simulink model "PreCondition"  (R2018b)
settings: Solver=FixedStepDiscrete  StartTime=0.0  StopTime=10.0  FixedStep=0.01  RelTol=1e-3
undefined symbols (not defined in the file or in its folder): EnergyMgLdShdRq1, HMI_2L_StMd10_Config_Val, HMI_2L_StMd11_Config_Val, HMI_2L_StMd12_Config_Val, HMI_2L_StMd13_Config_Val, HMI_2L_StMd14_Config_Val, HMI_2L_StMd15_Config_Val, HMI_2L_StMd16_Config_Val, HMI_2L_StMd17_Config_Val, HMI_2L_StMd18_Config_Val, HMI_2L_StMd19_Config_Val, HMI_2L_StMd1_Config_Val, HMI_2L_StMd20_Config_Val, HMI_2L_StMd21_Config_Val, HMI_2L_StMd22_Config_Val, HMI_2L_StMd23_Config_Val, HMI_2L_StMd24_Config_Val, HMI_2L_StMd25_Config_Val, HMI_2L_StMd26_Config_Val, HMI_2L_StMd27_Config_Val, HMI_2L_StMd28_Config_Val, HMI_2L_StMd29_Config_Val, HMI_2L_StMd2_Config_Val, HMI_2L_StMd30_Config_Val, HMI_2L_StMd31_Config_Val, HMI_2L_StMd32_Config_Val, HMI_2L_StMd3_Config_Val, HMI_2L_StMd4_Config_Val, HMI_2L_StMd5_Config_Val, HMI_2L_StMd6_Config_Val, HMI_2L_StMd7_Config_Val, HMI_2L_StMd8_Config_Val, HMI_2L_StMd9_Config_Val, HMI_2R_StMd10_Config_Val, HMI_2R_StMd11_Config_Val, HMI_2R_StMd12_Config_Val, HMI_2R_StMd13_Config_Val, HMI_2R_StMd14_Config_Val, HMI_2R_StMd15_Config_Val, HMI_2R_StMd16_Config_Val, HMI_2R_StMd17_Config_Val, HMI_2R_StMd18_Config_Val, HMI_2R_StMd19_Config_Val, HMI_2R_StMd1_Config_Val, HMI_2R_StMd20_Config_Val, HMI_2R_StMd21_Config_Val, HMI_2R_StMd22_Config_Val, HMI_2R_StMd23_Config_Val, HMI_2R_StMd24_Config_Val, HMI_2R_StMd25_Config_Val, HMI_2R_StMd26_Config_Val, HMI_2R_StMd27_Config_Val, HMI_2R_StMd28_Config_Val, HMI_2R_StMd29_Config_Val, HMI_2R_StMd2_Config_Val, HMI_2R_StMd30_Config_Val, HMI_2R_StMd31_Config_Val, HMI_2R_StMd32_Config_Val, HMI_2R_StMd3_Config_Val, HMI_2R_StMd4_Config_Val ... (+94)
(part 5 of 6)

== system PreCondition/PreConitionRunnable_sys/Subsystem3/AcsEntry4s2LMd ==
  CommCond : Inport
  AcsEntry4s2LMdConfig : Inport  Port=2
  SecRwLtStChldLkReq : Inport  Port=3
  AcsEntry4s2LPosLrnd : Inport  Port=4
  Is2LStSwAct : Inport  Port=5
  SecRwLtStPosRclRspStat : Inport  Port=6
  AND : Logic  Inputs=6  AllPortsSameDT=off  OutDataTypeStr=boolean
  Constant1 : Constant  Value=SeatChldLkSt.ChldLkSt_Unlock  OutDataTypeStr=Enum:SeatChldLkSt
  Constant4 : Constant  Value=PosRclRspStat1.PosRclRspStat_None  OutDataTypeStr=Enum:PosRclRspStat1
  Equal : RelationalOperator  Operator===  OutDataTypeStr=boolean  RndMeth=Simplest
  Equal5 : RelationalOperator  Operator===  OutDataTypeStr=boolean  RndMeth=Simplest
  NOT : Logic  Operator=NOT  AllPortsSameDT=off  OutDataTypeStr=boolean
  "AcsEntry4s2LAvl " : Outport
  wires:
  CommCond/1 -> AND/1
  AcsEntry4s2LMdConfig/1 -> AND/2
  AND/1 -> "AcsEntry4s2LAvl "/1
  AcsEntry4s2LPosLrnd/1 -> AND/4
  NOT/1 -> AND/5
  Is2LStSwAct/1 -> NOT/1
  Constant1/1 -> Equal5/2
  SecRwLtStChldLkReq/1 -> Equal5/1
  Equal5/1 -> AND/3
  Constant4/1 -> Equal/2
  [SecRwLtStPosRclRspStat] -> Equal/1
  Equal/1 -> AND/6
  SecRwLtStPosRclRspStat/1 -> [SecRwLtStPosRclRspStat]

== system PreCondition/PreConitionRunnable_sys/Subsystem3/AcsEntry4s2RMd ==
  CommCond : Inport
  AcsEntry4s2RMdConfig : Inport  Port=2
  SecRwRtStChldLkReq : Inport  Port=3
  AcsEntry4s2RPosLrnd : Inport  Port=4
  Is2RStSwAct : Inport  Port=5
  VeSignalLost2R_463_2L : Inport  Port=6
  SecRwRtStPosRclRspStat : Inport  Port=7
  AND : Logic  Inputs=7  AllPortsSameDT=off  OutDataTypeStr=boolean
  Constant3 : Constant  Value=SeatChldLkSt.ChldLkSt_Unlock  OutDataTypeStr=Enum:SeatChldLkSt
  Constant4 : Constant  Value=PosRclRspStat1.PosRclRspStat_None  OutDataTypeStr=Enum:PosRclRspStat1
  Equal : RelationalOperator  Operator===  OutDataTypeStr=boolean  RndMeth=Simplest
  Equal2 : RelationalOperator  Operator===  OutDataTypeStr=boolean  RndMeth=Simplest
  NOT : Logic  Operator=NOT  AllPortsSameDT=off  OutDataTypeStr=boolean
  NOT1 : Logic  Operator=NOT  AllPortsSameDT=off  OutDataTypeStr=boolean
  "AcsEntry4s2RAvl " : Outport
  wires:
  CommCond/1 -> AND/1
  AcsEntry4s2RMdConfig/1 -> AND/2
  AND/1 -> "AcsEntry4s2RAvl "/1
  AcsEntry4s2RPosLrnd/1 -> AND/4
  NOT/1 -> AND/5
  Is2RStSwAct/1 -> NOT/1
  VeSignalLost2R_463_2L/1 -> NOT1/1
  NOT1/1 -> AND/6
  Equal2/1 -> AND/3
  SecRwRtStChldLkReq/1 -> Equal2/1
  Constant3/1 -> Equal2/2
  Constant4/1 -> Equal/2
  [SecRwRtStPosRclRspStat] -> Equal/1
  Equal/1 -> AND/7
  SecRwRtStPosRclRspStat/1 -> [SecRwRtStPosRclRspStat]

== system PreCondition/PreConitionRunnable_sys/Subsystem3/AcsEntryAll4sBwdMd ==
  CommCond : Inport
  AcsEntryAll4sBwdMdConfig : Inport  Port=2
  SecRwLtStChldLkReq : Inport  Port=3
  SecRwRtStChldLkReq : Inport  Port=4
  AcsEntryAll4sBwdPosLrnd : Inport  Port=5
  Is2LStSwAct : Inport  Port=6
  Is2RStSwAct : Inport  Port=7
  VeSignalLost2R_463_2L : Inport  Port=8
  SecRwLtStPosRclRspStat : Inport  Port=9
  SecRwRtStPosRclRspStat : Inport  Port=10
  AND : Logic  Inputs=7  AllPortsSameDT=off  OutDataTypeStr=boolean
  AND1 : Logic  AllPortsSameDT=off  OutDataTypeStr=boolean
  AND2 : Logic  AllPortsSameDT=off  OutDataTypeStr=boolean
  Constant1 : Constant  Value=SeatChldLkSt.ChldLkSt_Unlock  OutDataTypeStr=Enum:SeatChldLkSt
  Constant2 : Constant  Value=PosRclRspStat1.PosRclRspStat_None  OutDataTypeStr=Enum:PosRclRspStat1
  Constant4 : Constant  Value=PosRclRspStat1.PosRclRspStat_None  OutDataTypeStr=Enum:PosRclRspStat1
  Equal{,1..2,5} (4 alike) : RelationalOperator  Operator===  OutDataTypeStr=boolean  RndMeth=Simplest
  NOT : Logic  Operator=NOT  AllPortsSameDT=off  OutDataTypeStr=boolean
  NOT1 : Logic  Operator=NOT  AllPortsSameDT=off  OutDataTypeStr=boolean
  OR : Logic  Operator=OR  AllPortsSameDT=off  OutDataTypeStr=boolean
  "AcsEntryAll4sBwdAvl " : Outport
  wires:
  OR/1 -> NOT/1
  Is2RStSwAct/1 -> OR/2
  Is2LStSwAct/1 -> OR/1
  Equal1/1 -> AND1/2
  SecRwRtStChldLkReq/1 -> Equal1/2
  SecRwLtStChldLkReq/1 -> Equal5/1
  Constant1/1 -> Equal5/2, Equal1/1
  AND1/1 -> AND/3
  Equal5/1 -> AND1/1
  NOT1/1 -> AND/6
  VeSignalLost2R_463_2L/1 -> NOT1/1
  NOT/1 -> AND/5
  AcsEntryAll4sBwdPosLrnd/1 -> AND/4
  AND/1 -> "AcsEntryAll4sBwdAvl "/1
  AcsEntryAll4sBwdMdConfig/1 -> AND/2
  CommCond/1 -> AND/1
  [SecRwRtStPosRclRspStat] -> Equal2/1
  Equal2/1 -> AND2/2
  Constant2/1 -> Equal2/2
  [SecRwLtStPosRclRspStat] -> Equal/1
  Constant4/1 -> Equal/2
  Equal/1 -> AND2/1
  AND2/1 -> AND/7
  SecRwLtStPosRclRspStat/1 -> [SecRwLtStPosRclRspStat]
  SecRwRtStPosRclRspStat/1 -> [SecRwRtStPosRclRspStat]

== system PreCondition/PreConitionRunnable_sys/Subsystem3/AcsEntryAll4sFwdMd ==
  CommCond : Inport
  AcsEntryAll4sFwdMdConfig : Inport  Port=2
  SecRwLtStChldLkReq : Inport  Port=3
  SecRwRtStChldLkReq : Inport  Port=4
  AcsEntryAll4sFwdPosLrnd : Inport  Port=5
  Is2LStSwAct : Inport  Port=6
  Is2RStSwAct : Inport  Port=7
  VeSignalLost2R_463_2L : Inport  Port=8
  SecRwLtStPosRclRspStat : Inport  Port=9
  SecRwRtStPosRclRspStat : Inport  Port=10
  AND : Logic  Inputs=7  AllPortsSameDT=off  OutDataTypeStr=boolean
  AND1 : Logic  AllPortsSameDT=off  OutDataTypeStr=boolean
  AND2 : Logic  AllPortsSameDT=off  OutDataTypeStr=boolean
  Constant1 : Constant  Value=SeatChldLkSt.ChldLkSt_Unlock  OutDataTypeStr=Enum:SeatChldLkSt
  Constant2 : Constant  Value=PosRclRspStat1.PosRclRspStat_None  OutDataTypeStr=Enum:PosRclRspStat1
  Constant4 : Constant  Value=PosRclRspStat1.PosRclRspStat_None  OutDataTypeStr=Enum:PosRclRspStat1
  Equal{,1..2,5} (4 alike) : RelationalOperator  Operator===  OutDataTypeStr=boolean  RndMeth=Simplest
  NOT : Logic  Operator=NOT  AllPortsSameDT=off  OutDataTypeStr=boolean
  NOT1 : Logic  Operator=NOT  AllPortsSameDT=off  OutDataTypeStr=boolean
  OR : Logic  Operator=OR  AllPortsSameDT=off  OutDataTypeStr=boolean
  "AcsEntryAll4sFwdAvl " : Outport
  wires:
  CommCond/1 -> AND/1
  AcsEntryAll4sFwdMdConfig/1 -> AND/2
  AND/1 -> "AcsEntryAll4sFwdAvl "/1
  AcsEntryAll4sFwdPosLrnd/1 -> AND/4
  NOT/1 -> AND/5
  VeSignalLost2R_463_2L/1 -> NOT1/1
  NOT1/1 -> AND/6
  Equal5/1 -> AND1/1
  AND1/1 -> AND/3
  Constant1/1 -> Equal1/1, Equal5/2
  SecRwLtStChldLkReq/1 -> Equal5/1
  SecRwRtStChldLkReq/1 -> Equal1/2
  Equal1/1 -> AND1/2
  Is2LStSwAct/1 -> OR/1
  Is2RStSwAct/1 -> OR/2
  OR/1 -> NOT/1
  Constant4/1 -> Equal/2
  [SecRwLtStPosRclRspStat] -> Equal/1
  Constant2/1 -> Equal2/2
  [SecRwRtStPosRclRspStat] -> Equal2/1
  Equal/1 -> AND2/1
  Equal2/1 -> AND2/2
  AND2/1 -> AND/7
  SecRwLtStPosRclRspStat/1 -> [SecRwLtStPosRclRspStat]
  SecRwRtStPosRclRspStat/1 -> [SecRwRtStPosRclRspStat]

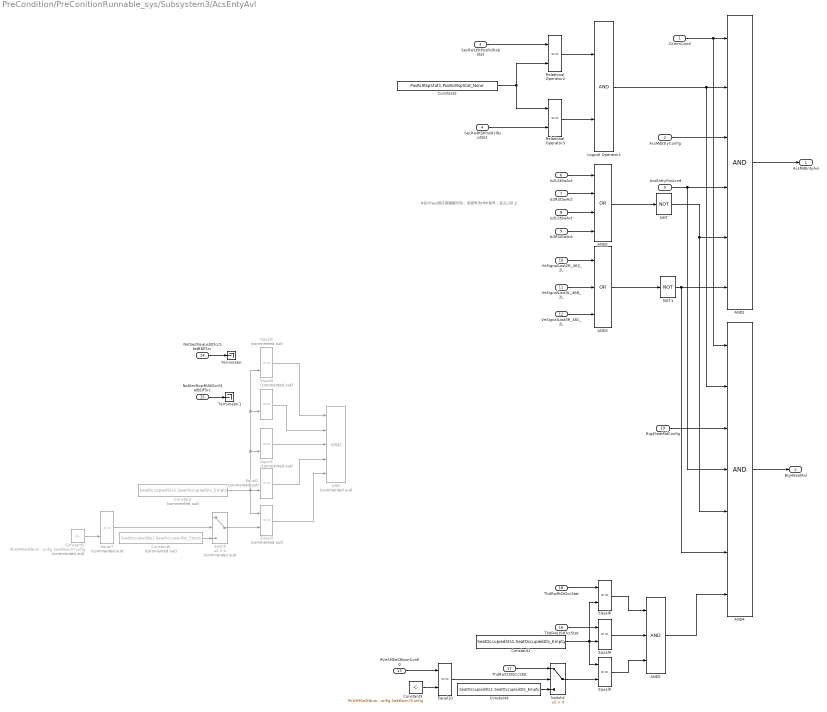
== system PreCondition/PreConitionRunnable_sys/Subsystem3/AcsEntyAvl ==
  note: #Dr/Pass侧只有脚蹬可动，该信号为HMI信号，在2L/2R上
  CommCond : Inport
  AcsMdEtryConfig : Inport  Port=2
  SecRwLtStPosRclRspStat : Inport  Port=3
  SecRwRtStPosRclRspStat : Inport  Port=4
  AcsEntryPosLrnd : Inport  Port=5
  Is2LStSwAct : Inport  Port=6
  Is2RStSwAct : Inport  Port=7
  Is3LStSwAct : Inport  Port=8
  Is3RStSwAct : Inport  Port=9
  VeSignalLost2R_463_2L : Inport  Port=10
  VeSignalLost3L_468_2L : Inport  Port=11
  VeSignalLost3R_46C_2L : Inport  Port=12
  IfVeSMSeStNumConfig : Inport  Port=13
  NotSecRowLeStOccStatBDFSrc : Inport  Port=14
  NotSecRowRtStOccStatBDFSrc : Inport  Port=15
  ThdRwLtStOccStat : Inport  Port=16
  ThdRwCtStOccStat : Inport  Port=17
  ThdRwRtStOccStat : Inport  Port=18
  Big4SeatMdConfig : Inport  Port=19
  AND : Logic  Commented=on  Inputs=5  AllPortsSameDT=off  OutDataTypeStr=boolean
  AND1 : Logic  Inputs=6  AllPortsSameDT=off  OutDataTypeStr=boolean
  AND2 : Logic  Operator=OR  Inputs=4  AllPortsSameDT=off  OutDataTypeStr=boolean
  AND3 : Logic  Operator=OR  Inputs=3  AllPortsSameDT=off  OutDataTypeStr=boolean
  AND4 : Logic  Inputs=7  AllPortsSameDT=off  OutDataTypeStr=boolean
  AND5 : Logic  Inputs=3  AllPortsSameDT=off  OutDataTypeStr=boolean
  Constant : Constant  Commented=on  Value=SeatOccupiedSts1.SeatOccupiedSts_Empty  OutDataTypeStr=Enum:SeatOccupiedSts1
  Constant1 : Constant  Value=SeatOccupiedSts1.SeatOccupiedSts_Empty  OutDataTypeStr=Enum:SeatOccupiedSts1
  Constant2 : Constant  Value=PosRclRspStat1.PosRclRspStat_None  OutDataTypeStr=Enum:PosRclRspStat1
  Constant3 : Constant  Value=IfVeSMSeStNumConfig.SeatNum7Config  OutDataTypeStr=Enum: IfVeSMSeStNumConfig
  Constant4 : Constant  Value=SeatOccupiedSts1.SeatOccupiedSts_Empty  OutDataTypeStr=Enum:SeatOccupiedSts1
  Constant5 : Constant  Commented=on  Value=IfVeSMSeStNumConfig.SeatNum7Config  OutDataTypeStr=Enum: IfVeSMSeStNumConfig
  Constant6 : Constant  Commented=on  Value=SeatOccupiedSts1.SeatOccupiedSts_Empty  OutDataTypeStr=Enum:SeatOccupiedSts1
  Equal{1..5,7} (6 alike) : RelationalOperator  Commented=on  Operator===  OutDataTypeStr=boolean  RndMeth=Simplest
  Equal{6,8..10} (4 alike) : RelationalOperator  Operator===  OutDataTypeStr=boolean  RndMeth=Simplest
  Logical Operator1 : Logic  AllPortsSameDT=off  OutDataTypeStr=boolean
  NOT : Logic  Operator=NOT  AllPortsSameDT=off  OutDataTypeStr=boolean
  NOT1 : Logic  Operator=NOT  AllPortsSameDT=off  OutDataTypeStr=boolean
  Relational Operator2 : RelationalOperator  Operator===  OutDataTypeStr=boolean  RndMeth=Simplest
  Relational Operator3 : RelationalOperator  Operator===  OutDataTypeStr=boolean  RndMeth=Simplest
  Switch : Switch  Commented=on  Criteria=u2 > Threshold
  Switch1 : Switch  Criteria=u2 > Threshold
  Terminator : Terminator
  Terminator1 : Terminator
  "AcsMdEntyAvl " : Outport
  Big4SeatAvl : Outport  Port=2
  wires:
  SecRwLtStPosRclRspStat/1 -> Relational Operator2/1
  Constant2/1 -> Relational Operator3/1, Relational Operator2/2
  Logical Operator1/1 -> AND4/2, AND1/2
  CommCond/1 -> AND4/1, AND1/1
  AcsMdEtryConfig/1 -> AND1/3
  AND1/1 -> "AcsMdEntyAvl "/1
  AND2/1 -> NOT/1
  AND3/1 -> NOT1/1
  AcsEntryPosLrnd/1 -> AND4/4, AND1/4
  NOT/1 -> AND4/5, AND1/5
  NOT1/1 -> AND4/6, AND1/6
  VeSignalLost2R_463_2L/1 -> AND3/1
  Relational Operator2/1 -> Logical Operator1/1
  Relational Operator3/1 -> Logical Operator1/2
  SecRwRtStPosRclRspStat/1 -> Relational Operator3/2
  Is2LStSwAct/1 -> AND2/1
  Is2RStSwAct/1 -> AND2/2
  Equal7/1 -> Switch/2
  Constant5/1 -> Equal7/2
  Constant/1 -> Equal5/2, Equal4/2, Equal1/2, Equal2/2, Equal3/1
  Constant6/1 -> Switch/3
  Switch/1 -> Equal3/2
  Equal1/1 -> AND/3
  Equal5/1 -> AND/1
  Equal4/1 -> AND/2
  Equal2/1 -> AND/4
  Equal3/1 -> AND/5
  VeSignalLost3R_46C_2L/1 -> AND3/3
  VeSignalLost3L_468_2L/1 -> AND3/2
  Is3RStSwAct/1 -> AND2/4
  Is3LStSwAct/1 -> AND2/3
  NotSecRowLeStOccStatBDFSrc/1 -> Terminator/1
  NotSecRowRtStOccStatBDFSrc/1 -> Terminator1/1
  Big4SeatMdConfig/1 -> AND4/3
  Equal10/1 -> Switch1/2
  Constant3/1 -> Equal10/2
  Constant1/1 -> Equal6/2, Equal8/2, Equal9/1
  Constant4/1 -> Switch1/3
  Switch1/1 -> Equal9/2
  IfVeSMSeStNumConfig/1 -> Equal10/1
  ThdRwCtStOccStat/1 -> Switch1/1
  ThdRwRtStOccStat/1 -> Equal6/1
  ThdRwLtStOccStat/1 -> Equal8/1
  Equal8/1 -> AND5/2
  Equal6/1 -> AND5/1
  Equal9/1 -> AND5/3
  AND5/1 -> AND4/7
  AND4/1 -> Big4SeatAvl/1

== system PreCondition/PreConitionRunnable_sys/Subsystem3/AcsExit4s2LMd ==
  CommCond : Inport
  AcsExit4s2LMdConfig : Inport  Port=2
  SecRwLtStChldLkReq : Inport  Port=3
  AcsExit4s2LPosLrnd : Inport  Port=4
  Is2LStSwAct : Inport  Port=5
  SecRwLtStPosRclRspStat : Inport  Port=6
  AND : Logic  Inputs=6  AllPortsSameDT=off  OutDataTypeStr=boolean
  Constant1 : Constant  Value=SeatChldLkSt.ChldLkSt_Unlock  OutDataTypeStr=Enum:SeatChldLkSt
  Constant4 : Constant  Value=PosRclRspStat1.PosRclRspStat_None  OutDataTypeStr=Enum:PosRclRspStat1
  Equal : RelationalOperator  Operator===  OutDataTypeStr=boolean  RndMeth=Simplest
  Equal5 : RelationalOperator  Operator===  OutDataTypeStr=boolean  RndMeth=Simplest
  NOT : Logic  Operator=NOT  AllPortsSameDT=off  OutDataTypeStr=boolean
  "AcsExit4s2LAvl " : Outport
  wires:
  Is2LStSwAct/1 -> NOT/1
  NOT/1 -> AND/5
  AcsExit4s2LPosLrnd/1 -> AND/4
  AND/1 -> "AcsExit4s2LAvl "/1
  AcsExit4s2LMdConfig/1 -> AND/2
  CommCond/1 -> AND/1
  SecRwLtStChldLkReq/1 -> Equal5/1
  Constant1/1 -> Equal5/2
  Equal5/1 -> AND/3
  [SecRwLtStPosRclRspStat] -> Equal/1
  Constant4/1 -> Equal/2
  Equal/1 -> AND/6
  SecRwLtStPosRclRspStat/1 -> [SecRwLtStPosRclRspStat]

== system PreCondition/PreConitionRunnable_sys/Subsystem3/AcsExit4s2RMd ==
  CommCond : Inport
  AcsExit4s2RMdConfig : Inport  Port=2
  SecRwRtStChldLkReq : Inport  Port=3
  AcsExit4s2RPosLrnd : Inport  Port=4
  Is2RStSwAct : Inport  Port=5
  VeSignalLost2R_463_2L : Inport  Port=6
  SecRwRtStPosRclRspStat : Inport  Port=7
  AND : Logic  Inputs=7  AllPortsSameDT=off  OutDataTypeStr=boolean
  Constant3 : Constant  Value=SeatChldLkSt.ChldLkSt_Unlock  OutDataTypeStr=Enum:SeatChldLkSt
  Constant4 : Constant  Value=PosRclRspStat1.PosRclRspStat_None  OutDataTypeStr=Enum:PosRclRspStat1
  Equal : RelationalOperator  Operator===  OutDataTypeStr=boolean  RndMeth=Simplest
  Equal2 : RelationalOperator  Operator===  OutDataTypeStr=boolean  RndMeth=Simplest
  NOT : Logic  Operator=NOT  AllPortsSameDT=off  OutDataTypeStr=boolean
  NOT1 : Logic  Operator=NOT  AllPortsSameDT=off  OutDataTypeStr=boolean
  "AcsExit4s2RAvl " : Outport
  wires:
  NOT1/1 -> AND/6
  VeSignalLost2R_463_2L/1 -> NOT1/1
  Is2RStSwAct/1 -> NOT/1
  NOT/1 -> AND/5
  AcsExit4s2RPosLrnd/1 -> AND/4
  AND/1 -> "AcsExit4s2RAvl "/1
  AcsExit4s2RMdConfig/1 -> AND/2
  CommCond/1 -> AND/1
  Constant3/1 -> Equal2/2
  SecRwRtStChldLkReq/1 -> Equal2/1
  Equal2/1 -> AND/3
  Constant4/1 -> Equal/2
  [SecRwRtStPosRclRspStat] -> Equal/1
  Equal/1 -> AND/7
  SecRwRtStPosRclRspStat/1 -> [SecRwRtStPosRclRspStat]

== system PreCondition/PreConitionRunnable_sys/Subsystem3/AcsExtAvl ==
  CommCond : Inport
  AcsMdExitConfig : Inport  Port=2
  SecRwLtStPosRclRspStat : Inport  Port=3
  SecRwRtStPosRclRspStat : Inport  Port=4
  AcsExitPosLrnd : Inport  Port=5
  IsDrvStSwAct : Inport  Port=6
  IsPasStSwAct : Inport  Port=7
  Is2LStSwAct : Inport  Port=8
  Is2RStSwAct : Inport  Port=9
  VeSignalLost2R_463_2L : Inport  Port=10
  AND : Logic  Inputs=6  AllPortsSameDT=off  OutDataTypeStr=boolean
  AND2 : Logic  Operator=OR  Inputs=4  AllPortsSameDT=off  OutDataTypeStr=boolean
  Constant2 : Constant  Value=PosRclRspStat1.PosRclRspStat_None  OutDataTypeStr=Enum:PosRclRspStat1
  Logical Operator1 : Logic  AllPortsSameDT=off  OutDataTypeStr=boolean
  NOT : Logic  Operator=NOT  AllPortsSameDT=off  OutDataTypeStr=boolean
  NOT1 : Logic  Operator=NOT  AllPortsSameDT=off  OutDataTypeStr=boolean
  Relational Operator2 : RelationalOperator  Operator===  OutDataTypeStr=boolean  RndMeth=Simplest
  Relational Operator3 : RelationalOperator  Operator===  OutDataTypeStr=boolean  RndMeth=Simplest
  AcsMdExtAvl : Outport
  wires:
  CommCond/1 -> AND/1
  Constant2/1 -> Relational Operator2/2, Relational Operator3/1
  SecRwLtStPosRclRspStat/1 -> Relational Operator2/1
  Logical Operator1/1 -> AND/3
  AcsMdExitConfig/1 -> AND/2
  AND/1 -> AcsMdExtAvl/1
  AND2/1 -> NOT/1
  Is2RStSwAct/1 -> AND2/4
  Is2LStSwAct/1 -> AND2/3
  IsDrvStSwAct/1 -> AND2/1
  IsPasStSwAct/1 -> AND2/2
  AcsExitPosLrnd/1 -> AND/4
  NOT/1 -> AND/5
  NOT1/1 -> AND/6
  Relational Operator2/1 -> Logical Operator1/1
  Relational Operator3/1 -> Logical Operator1/2
  VeSignalLost2R_463_2L/1 -> NOT1/1
  SecRwRtStPosRclRspStat/1 -> Relational Operator3/2

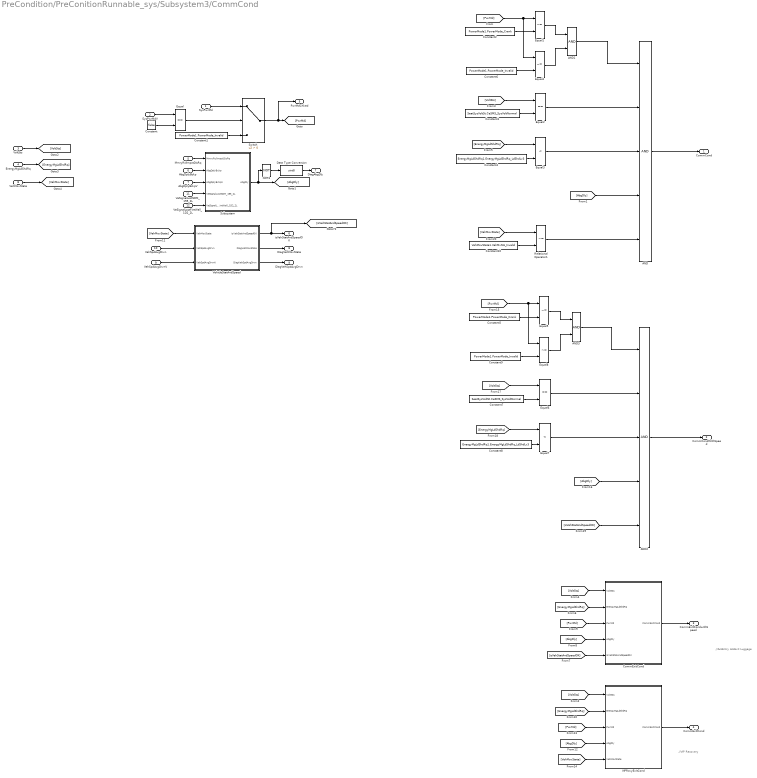
== system PreCondition/PreConitionRunnable_sys/Subsystem3/CommCond  ==
  note: //AcsEntry AcsExit Luggage
  note: //VIP Recovery
  SysPwrMd : Inport
  SysPwrMdV : Inport  Port=2
  VoltSts : Inport  Port=3
  EnergyMgLdShdRq : Inport  Port=4
  MmryRclImpctDisRq : Inport  Port=5
  AbgDplyBckp : Inport  Port=6
  AbgDplyBckpV : Inport  Port=7
  VehMovState : Inport  Port=8
  VehSpdAvgDrvnV : Inport  Port=9
  VehSpdAvgDrvn : Inport  Port=10
  VeSignalLostSDM_195_2L : Inport  Port=11
  VeSignalLostFireWall_1D2_2L : Inport  Port=12
  " VehicleStatAndSpeed" : Subsystem
  AND : Logic  Inputs=5  AllPortsSameDT=off  OutDataTypeStr=boolean
  AND1 : Logic  AllPortsSameDT=off  OutDataTypeStr=boolean
  AND2 : Logic  Inputs=5  AllPortsSameDT=off  OutDataTypeStr=boolean
  AND3 : Logic  AllPortsSameDT=off  OutDataTypeStr=boolean
  "CommExitCond " : Subsystem
  Constant : Constant  Value=false  OutDataTypeStr=boolean
  Constant1 : Constant  Value=PowerMode1.PowerMode_Invalid
  Constant10 : Constant  Value=VehMovState1.VehMvSts_Invalid  OutDataTypeStr=Enum:VehMovState1
  Constant2 : Constant  Value=PowerMode1.PowerMode_Crank
  Constant3 : Constant  Value=SeatSysVoltSt.CeSMS_SysVoltNormal
  Constant4 : Constant  Value=EnergyMgLdShdRq1.EnergyMgLdShdRq_LdShdLv3
  Constant5 : Constant  Value=PowerMode1.PowerMode_Crank
  Constant6 : Constant  Value=PowerMode1.PowerMode_Invalid
  Constant7 : Constant  Value=SeatSysVoltSt.CeSMS_SysVoltNormal
  Constant8 : Constant  Value=EnergyMgLdShdRq1.EnergyMgLdShdRq_LdShdLv3
  Constant9 : Constant  Value=PowerMode1.PowerMode_Invalid
  Data Type Conversion : DataTypeConversion  OutDataTypeStr=uint8
  Equal : RelationalOperator  Operator===  OutDataTypeStr=boolean  RndMeth=Simplest
  Equal{1,4..5,8} (4 alike) : RelationalOperator  Operator=~=  OutDataTypeStr=boolean  RndMeth=Simplest
  Equal2 : RelationalOperator  Operator===  OutDataTypeStr=boolean  RndMeth=Simplest
  Equal3 : RelationalOperator  Operator=<  OutDataTypeStr=boolean  RndMeth=Simplest
  Equal6 : RelationalOperator  Operator===  OutDataTypeStr=boolean  RndMeth=Simplest
  Equal7 : RelationalOperator  Operator=<  OutDataTypeStr=boolean  RndMeth=Simplest
  NOT3 : Logic  Operator=NOT  AllPortsSameDT=off  OutDataTypeStr=boolean
  Relational Operator1 : RelationalOperator  Operator=~=  OutDataTypeStr=boolean  RndMeth=Simplest
  Subsystem : Subsystem
  Switch : Switch  Criteria=u2 > Threshold
  "VIPRcvyExitCond " : Subsystem
  "CommCond " : Outport
  "CommCondWithSpeed " : Outport  Port=2
  CommExitCondwithSpeed : Outport  Port=3
  CommExitCond : Outport  Port=4
  PwrMdChked : Outport  Port=5
  isVehStatAndSpeedOK : Outport  Port=6
  DiagAbgDly : Outport  Port=7
  DiagVehMovState : Outport  Port=8
  DiagVehSpdAvgDrvn : Outport  Port=9
  wires:
  SysPwrMdV/1 -> Equal/1
  Equal/1 -> Switch/2
  Constant/1 -> Equal/2
  Constant2/1 -> Equal1/2
  [PwrMd] -> Equal4/1, Equal1/1
  SysPwrMd/1 -> Switch/1
  Switch/1 -> PwrMdChked/1, [PwrMd]
  Constant1/1 -> Switch/3
  Constant3/1 -> Equal2/2
  Equal2/1 -> AND/2
  AND/1 -> "CommCond "/1
  Constant4/1 -> Equal3/2
  Equal3/1 -> AND/3
  MmryRclImpctDisRq/1 -> Subsystem/1(MmryRclImpctDisRq)
  AbgDplyBckp/1 -> Subsystem/2(AbgDplyBckp)
  AbgDplyBckpV/1 -> Subsystem/3(AbgDplyBckpV)
  Subsystem/1(AbgDly) -> NOT3/1, [AbgDly]
  [AbgDly] -> AND/4
  VehSpdAvgDrvn/1 -> " VehicleStatAndSpeed"/2(VehSpdAvgDrvn)
  VehSpdAvgDrvnV/1 -> " VehicleStatAndSpeed"/3(VehSpdAvgDrvnV)
  " VehicleStatAndSpeed"/1(isVehStatAndSpeedOK) -> isVehStatAndSpeedOK/1, [isVehStatAndSpeedOK]
  "CommExitCond "/1("CommExitCond ") -> CommExitCondwithSpeed/1
  VoltSts/1 -> [VoltSts]
  [VoltSts] -> Equal2/1
  [VoltSts] -> "CommExitCond "/1(VoltSts)
  EnergyMgLdShdRq/1 -> [EnergyMgLdShdRq]
  [EnergyMgLdShdRq] -> Equal3/1
  [EnergyMgLdShdRq] -> "CommExitCond "/2(EnergyMgLdShdRq)
  [AbgDly] -> "CommExitCond "/4(AbgDly)
  [PwrMd] -> "CommExitCond "/3(PwrMd)
  [isVehStatAndSpeedOK] -> "CommExitCond "/5(isVehStatAndSpeedOK)
  [VoltSts] -> "VIPRcvyExitCond "/1(VoltSts)
  [PwrMd] -> "VIPRcvyExitCond "/3(PwrMd)
  [EnergyMgLdShdRq] -> "VIPRcvyExitCond "/2(EnergyMgLdShdRq)
  "VIPRcvyExitCond "/1("CommExitCond ") -> CommExitCond/1
  [AbgDly] -> "VIPRcvyExitCond "/4(AbgDly)
  Constant6/1 -> Equal4/2
  Equal1/1 -> AND1/1
  Equal4/1 -> AND1/2
  AND1/1 -> AND/1
  VeSignalLostSDM_195_2L/1 -> Subsystem/4(VeSignalLostSDM_195_2L)
  VeSignalLostFireWall_1D2_2L/1 -> Subsystem/5(VeSignalLostFireWall_1D2_2L)
  VehMovState/1 -> [VehMovState]
  [VehMovState] -> " VehicleStatAndSpeed"/1(VehMovState)
  [VehMovState] -> "VIPRcvyExitCond "/5(VehMovState)
  Equal8/1 -> AND3/2
  AND3/1 -> AND2/1
  [PwrMd] -> Equal8/1, Equal5/1
  Constant9/1 -> Equal8/2
  AND2/1 -> "CommCondWithSpeed "/1
  Equal5/1 -> AND3/1
  [VoltSts] -> Equal6/1
  [EnergyMgLdShdRq] -> Equal7/1
  [AbgDly] -> AND2/4
  Constant8/1 -> Equal7/2
  Equal7/1 -> AND2/3
  Constant5/1 -> Equal5/2
  Equal6/1 -> AND2/2
  Constant7/1 -> Equal6/2
  [isVehStatAndSpeedOK] -> AND2/5
  [VehMovState] -> Relational Operator1/1
  Constant10/1 -> Relational Operator1/2
  Relational Operator1/1 -> AND/5
  " VehicleStatAndSpeed"/2(DiagVehMovState) -> DiagVehMovState/1
  " VehicleStatAndSpeed"/3(DiagVehSpdAvgDrvn) -> DiagVehSpdAvgDrvn/1
  NOT3/1 -> Data Type Conversion/1
  Data Type Conversion/1 -> DiagAbgDly/1

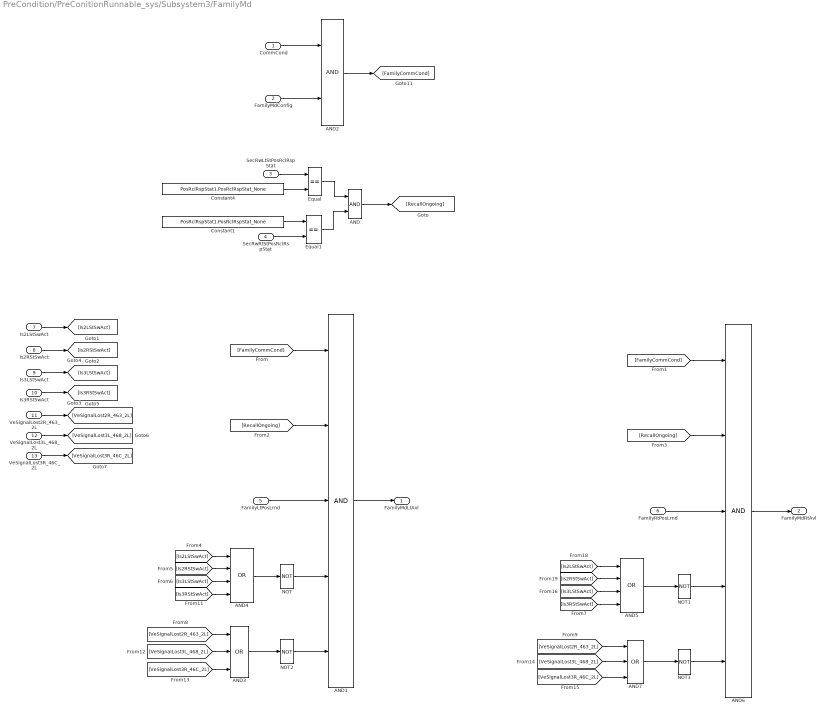
== system PreCondition/PreConitionRunnable_sys/Subsystem3/FamilyMd ==
  CommCond : Inport
  FamilyMdConfig : Inport  Port=2
  SecRwLtStPosRclRspStat : Inport  Port=3
  SecRwRtStPosRclRspStat : Inport  Port=4
  FamilyLtPosLrnd : Inport  Port=5
  FamilyRtPosLrnd : Inport  Port=6
  Is2LStSwAct : Inport  Port=7
  Is2RStSwAct : Inport  Port=8
  Is3LStSwAct : Inport  Port=9
  Is3RStSwAct : Inport  Port=10
  VeSignalLost2R_463_2L : Inport  Port=11
  VeSignalLost3L_468_2L : Inport  Port=12
  VeSignalLost3R_46C_2L : Inport  Port=13
  AND : Logic  AllPortsSameDT=off  OutDataTypeStr=boolean
  AND1 : Logic  Inputs=5  AllPortsSameDT=off  OutDataTypeStr=boolean
  AND2 : Logic  AllPortsSameDT=off  OutDataTypeStr=boolean
  AND3 : Logic  Operator=OR  Inputs=3  AllPortsSameDT=off  OutDataTypeStr=boolean
  AND4 : Logic  Operator=OR  Inputs=4  AllPortsSameDT=off  OutDataTypeStr=boolean
  AND5 : Logic  Operator=OR  Inputs=4  AllPortsSameDT=off  OutDataTypeStr=boolean
  AND6 : Logic  Inputs=5  AllPortsSameDT=off  OutDataTypeStr=boolean
  AND7 : Logic  Operator=OR  Inputs=3  AllPortsSameDT=off  OutDataTypeStr=boolean
  Constant1 : Constant  Value=PosRclRspStat1.PosRclRspStat_None  OutDataTypeStr=Enum:PosRclRspStat1
  Constant4 : Constant  Value=PosRclRspStat1.PosRclRspStat_None  OutDataTypeStr=Enum:PosRclRspStat1
  Equal : RelationalOperator  Operator===  OutDataTypeStr=boolean  RndMeth=Simplest
  Equal1 : RelationalOperator  Operator===  OutDataTypeStr=boolean  RndMeth=Simplest
  NOT{,1..3} (4 alike) : Logic  Operator=NOT  AllPortsSameDT=off  OutDataTypeStr=boolean
  FamilyMdLtAvl : Outport
  FamilyMdRtAvl : Outport  Port=2
  wires:
  CommCond/1 -> AND2/1
  AND2/1 -> [FamilyCommCond]
  FamilyMdConfig/1 -> AND2/2
  NOT2/1 -> AND1/5
  AND1/1 -> FamilyMdLtAvl/1
  Equal1/1 -> AND/2
  SecRwLtStPosRclRspStat/1 -> Equal/1
  [FamilyCommCond] -> AND1/1
  SecRwRtStPosRclRspStat/1 -> Equal1/2
  Constant1/1 -> Equal1/1
  Equal/1 -> AND/1
  AND4/1 -> NOT/1
  Constant4/1 -> Equal/2
  NOT/1 -> AND1/4
  FamilyLtPosLrnd/1 -> AND1/3
  AND3/1 -> NOT2/1
  AND7/1 -> NOT3/1
  [VeSignalLost2R_463_2L] -> AND7/1
  AND5/1 -> NOT1/1
  NOT1/1 -> AND6/4
  FamilyRtPosLrnd/1 -> AND6/3
  NOT3/1 -> AND6/5
  [FamilyCommCond] -> AND6/1
  AND6/1 -> FamilyMdRtAvl/1
  AND/1 -> [RecallOngoing]
  [RecallOngoing] -> AND1/2
  [RecallOngoing] -> AND6/2
  Is2LStSwAct/1 -> [Is2LStSwAct]
  Is2RStSwAct/1 -> [Is2RStSwAct]
  [Is2LStSwAct] -> AND4/1
  [Is2RStSwAct] -> AND4/2
  VeSignalLost2R_463_2L/1 -> [VeSignalLost2R_463_2L]
  [VeSignalLost2R_463_2L] -> AND3/1
  Is3LStSwAct/1 -> [Is3LStSwAct]
  Is3RStSwAct/1 -> [Is3RStSwAct]
  VeSignalLost3L_468_2L/1 -> [VeSignalLost3L_468_2L]
  VeSignalLost3R_46C_2L/1 -> [VeSignalLost3R_46C_2L]
  [VeSignalLost3L_468_2L] -> AND3/2
  [VeSignalLost3R_46C_2L] -> AND3/3
  [VeSignalLost3L_468_2L] -> AND7/2
  [VeSignalLost3R_46C_2L] -> AND7/3
  [Is3LStSwAct] -> AND5/3
  [Is2RStSwAct] -> AND5/2
  [Is2LStSwAct] -> AND5/1
  [Is3RStSwAct] -> AND4/4
  [Is3LStSwAct] -> AND4/3
  [Is3RStSwAct] -> AND5/4

== system PreCondition/PreConitionRunnable_sys/Subsystem3/IntimacyMd ==
  CommCond : Inport
  IntimacyMdConfig : Inport  Port=2
  SecRwLtStPosRclRspStat : Inport  Port=3
  SecRwRtStPosRclRspStat : Inport  Port=4
  IntimacyLPosLrnd : Inport  Port=5
  IntimacyRPosLrnd : Inport  Port=6
  Is2LStSwAct : Inport  Port=7
  Is2RStSwAct : Inport  Port=8
  VeSignalLost2R_463_2L : Inport  Port=9
  AND : Logic  AllPortsSameDT=off  OutDataTypeStr=boolean
  AND1 : Logic  Inputs=5  AllPortsSameDT=off  OutDataTypeStr=boolean
  AND2 : Logic  AllPortsSameDT=off  OutDataTypeStr=boolean
  AND3 : Logic  AllPortsSameDT=off  OutDataTypeStr=boolean
  AND4 : Logic  Operator=OR  AllPortsSameDT=off  OutDataTypeStr=boolean
  AND5 : Logic  Inputs=5  AllPortsSameDT=off  OutDataTypeStr=boolean
  AND6 : Logic  Operator=OR  AllPortsSameDT=off  OutDataTypeStr=boolean
  Constant{1..4} (4 alike) : Constant  Value=PosRclRspStat1.PosRclRspStat_None  OutDataTypeStr=Enum:PosRclRspStat1
  Equal{,1..3} (4 alike) : RelationalOperator  Operator===  OutDataTypeStr=boolean  RndMeth=Simplest
  NOT{,1..3} (4 alike) : Logic  Operator=NOT  AllPortsSameDT=off  OutDataTypeStr=boolean
  IntimacyLMdAvl : Outport
  IntimacyRMdAvl : Outport  Port=2
  wires:
  AND2/1 -> [IntimacyCommCond]
  IntimacyMdConfig/1 -> AND2/2
  CommCond/1 -> AND2/1
  AND4/1 -> NOT/1
  IntimacyLPosLrnd/1 -> AND1/3
  NOT2/1 -> AND1/5
  AND1/1 -> IntimacyLMdAvl/1
  Constant4/1 -> Equal/2
  [IntimacyCommCond] -> AND1/1
  Constant1/1 -> Equal1/1
  Equal/1 -> AND/1
  Equal1/1 -> AND/2
  AND/1 -> AND1/2
  NOT/1 -> AND1/4
  Equal2/1 -> AND3/1
  AND3/1 -> AND5/2
  Equal3/1 -> AND3/2
  AND5/1 -> IntimacyRMdAvl/1
  Constant2/1 -> Equal3/1
  NOT1/1 -> AND5/4
  NOT3/1 -> AND5/5
  [IntimacyCommCond] -> AND5/1
  Constant3/1 -> Equal2/2
  IntimacyRPosLrnd/1 -> AND5/3
  AND6/1 -> NOT1/1
  SecRwLtStPosRclRspStat/1 -> [SecRwLtStPosRclRspStat]
  SecRwRtStPosRclRspStat/1 -> [SecRwRtStPosRclRspStat]
  [SecRwLtStPosRclRspStat] -> Equal/1
  [SecRwRtStPosRclRspStat] -> Equal1/2
  [SecRwLtStPosRclRspStat] -> Equal2/1
  [SecRwRtStPosRclRspStat] -> Equal3/2
  Is2LStSwAct/1 -> [Is2LStSwAct]
  Is2RStSwAct/1 -> [Is2RStSwAct]
  [Is2LStSwAct] -> AND4/1
  [Is2RStSwAct] -> AND4/2
  [Is2LStSwAct] -> AND6/1
  [Is2RStSwAct] -> AND6/2
  VeSignalLost2R_463_2L/1 -> [VeSignalLost2R_463_2L]
  [VeSignalLost2R_463_2L] -> NOT2/1
  [VeSignalLost2R_463_2L] -> NOT3/1

== system PreCondition/PreConitionRunnable_sys/Subsystem3/LgrstOpenLtMd ==
  CommCond : Inport
  LgrstLtMdConfig : Inport  Port=2
  SecRwLtStPosRclRspStat : Inport  Port=3
  LgrstOpenLtPosLrnd : Inport  Port=4
  LgrstCloseLtPosLrnd : Inport  Port=5
  Is2LStSwAct : Inport  Port=6
  AND1 : Logic  Inputs=4  AllPortsSameDT=off  OutDataTypeStr=boolean
  AND2 : Logic  AllPortsSameDT=off  OutDataTypeStr=boolean
  AND3 : Logic  Inputs=4  AllPortsSameDT=off  OutDataTypeStr=boolean
  Constant1 : Constant  Value=PosRclRspStat1.PosRclRspStat_None  OutDataTypeStr=Enum:PosRclRspStat1
  Constant4 : Constant  Value=PosRclRspStat1.PosRclRspStat_None  OutDataTypeStr=Enum:PosRclRspStat1
  Equal : RelationalOperator  Operator===  OutDataTypeStr=boolean  RndMeth=Simplest
  Equal1 : RelationalOperator  Operator===  OutDataTypeStr=boolean  RndMeth=Simplest
  NOT : Logic  Operator=NOT  AllPortsSameDT=off  OutDataTypeStr=boolean
  NOT1 : Logic  Operator=NOT  AllPortsSameDT=off  OutDataTypeStr=boolean
  LgrstOpenLtMdAvl : Outport
  LgrstCloseLtMdAvl : Outport  Port=2
  wires:
  AND2/1 -> [LgrstLtCommCond]
  CommCond/1 -> AND2/1
  LgrstLtMdConfig/1 -> AND2/2
  LgrstOpenLtPosLrnd/1 -> AND1/3
  NOT/1 -> AND1/4
  Constant4/1 -> Equal/2
  AND1/1 -> LgrstOpenLtMdAvl/1
  Equal/1 -> AND1/2
  [LgrstLtCommCond] -> AND1/1
  NOT1/1 -> AND3/4
  [LgrstLtCommCond] -> AND3/1
  AND3/1 -> LgrstCloseLtMdAvl/1
  Equal1/1 -> AND3/2
  Constant1/1 -> Equal1/2
  [SecRwLtStPosRclRspStat] -> Equal1/1
  LgrstCloseLtPosLrnd/1 -> AND3/3
  [Is2LStSwAct] -> NOT1/1
  SecRwLtStPosRclRspStat/1 -> [SecRwLtStPosRclRspStat]
  [SecRwLtStPosRclRspStat] -> Equal/1
  Is2LStSwAct/1 -> [Is2LStSwAct]
  [Is2LStSwAct] -> NOT/1

== system PreCondition/PreConitionRunnable_sys/Subsystem3/LgrstOpenRtMd ==
  CommCond : Inport
  LgrstRtMdConfig : Inport  Port=2
  SecRwRtStPosRclRspStat : Inport  Port=3
  LgrstOpenRtPosLrnd : Inport  Port=4
  LgrstCloseRtPosLrnd : Inport  Port=5
  Is2RStSwAct : Inport  Port=6
  VeSignalLost2R_463_2L : Inport  Port=7
  AND1 : Logic  Inputs=5  AllPortsSameDT=off  OutDataTypeStr=boolean
  AND2 : Logic  AllPortsSameDT=off  OutDataTypeStr=boolean
  AND3 : Logic  Inputs=5  AllPortsSameDT=off  OutDataTypeStr=boolean
  Constant1 : Constant  Value=PosRclRspStat1.PosRclRspStat_None  OutDataTypeStr=Enum:PosRclRspStat1
  Constant4 : Constant  Value=PosRclRspStat1.PosRclRspStat_None  OutDataTypeStr=Enum:PosRclRspStat1
  Equal : RelationalOperator  Operator===  OutDataTypeStr=boolean  RndMeth=Simplest
  Equal1 : RelationalOperator  Operator===  OutDataTypeStr=boolean  RndMeth=Simplest
  NOT{,1..3} (4 alike) : Logic  Operator=NOT  AllPortsSameDT=off  OutDataTypeStr=boolean
  LgrstOpenRtMdAvl : Outport
  LgrstCloseRtMdAvl : Outport  Port=2
  wires:
  AND2/1 -> [LgrstRtCommCond]
  CommCond/1 -> AND2/1
  LgrstRtMdConfig/1 -> AND2/2
  LgrstOpenRtPosLrnd/1 -> AND1/3
  NOT/1 -> AND1/4
  Constant4/1 -> Equal/2
  AND1/1 -> LgrstOpenRtMdAvl/1
  Equal/1 -> AND1/2
  [LgrstRtCommCond] -> AND1/1
  NOT2/1 -> AND1/5
  AND3/1 -> LgrstCloseRtMdAvl/1
  LgrstCloseRtPosLrnd/1 -> AND3/3
  NOT3/1 -> AND3/5
  [SecRwRtStPosRclRspStat] -> Equal1/1
  [Is2RStSwAct] -> NOT1/1
  [LgrstRtCommCond] -> AND3/1
  Equal1/1 -> AND3/2
  NOT1/1 -> AND3/4
  Constant1/1 -> Equal1/2
  [VeSignalLost2R_463_2L] -> NOT3/1
  SecRwRtStPosRclRspStat/1 -> [SecRwRtStPosRclRspStat]
  [SecRwRtStPosRclRspStat] -> Equal/1
  Is2RStSwAct/1 -> [Is2RStSwAct]
  VeSignalLost2R_463_2L/1 -> [VeSignalLost2R_463_2L]
  [Is2RStSwAct] -> NOT/1
  [VeSignalLost2R_463_2L] -> NOT2/1

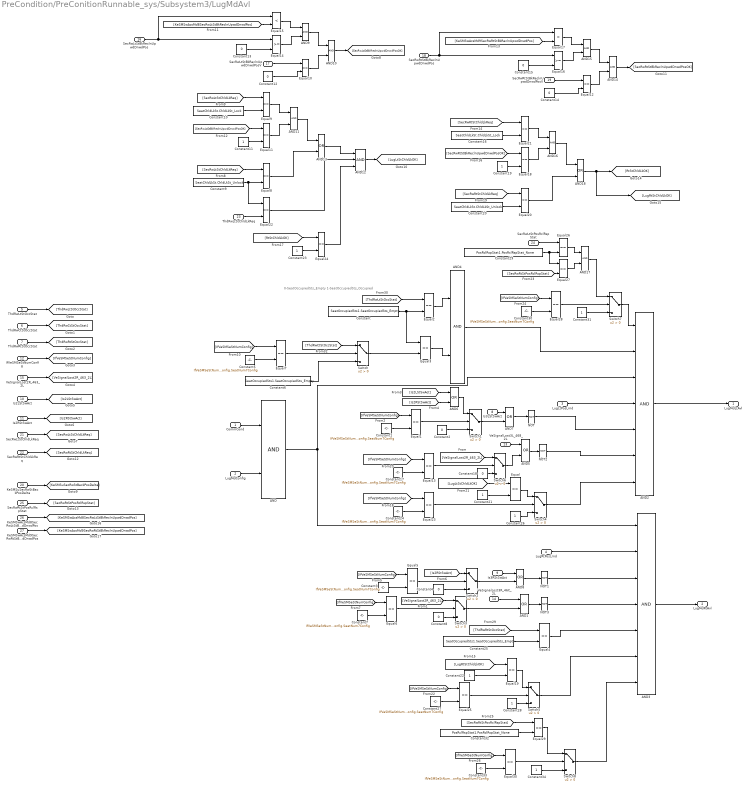
== system PreCondition/PreConitionRunnable_sys/Subsystem3/LugMdAvl ==
  note: 0-SeatOccupiedSts_Empty 1-SeatOccupiedSts_Occupied
  CommCond : Inport
  LugMdConfig : Inport  Port=2
  LugLtPosLrnd : Inport  Port=3
  LugRtPosLrnd : Inport  Port=4
  ThdRwLtStOccStat : Inport  Port=5
  ThdRwCtStOccStat : Inport  Port=6
  ThdRwRtStOccStat : Inport  Port=7
  Is3LStSwAct : Inport  Port=8
  Is3RStSwAct : Inport  Port=9
  Is2LStSwAct : Inport  Port=10
  Is2RStSwAct : Inport  Port=11
  IfVeSMSeStNumConfig : Inport  Port=12
  VeSignalLost3L_468_2L : Inport  Port=13
  VeSignalLost3R_46C_2L : Inport  Port=14
  VeSignalLost2R_463_2L : Inport  Port=15
  SecRwLtStBkReclnUpwdDnwdPos : Inport  Port=16
  SecRwLtStBkReclnUpwdDnwdPosV : Inport  Port=17
  SecRwRtStBkReclnUpwdDnwdPos : Inport  Port=18
  SecRwRtStBkReclnUpwdDnwdPosV : Inport  Port=19
  KeSMSuSecRwStBackPosDelta : Inport  Port=20
  SecRwLtStChldLkReq : Inport  Port=21
  SecRwRtStChldLkReq : Inport  Port=22
  ThdRwLtStChldLkReq : Inport  Port=23
  SecRwLtStPosRclRspStat : Inport  Port=24
  SecRwRtStPosRclRspStat : Inport  Port=25
  KeSMSwAcsMd8SecRwLtStBkReclnUpwdDnwdPos : Inport  Port=26
  KeSMSwAcsMd9SecRwRtStBkReclnUpwdDnwdPos : Inport  Port=27
  AND{,4,9..11,14..17} (9 alike) : Logic  AllPortsSameDT=off  OutDataTypeStr=boolean
  AND{1,5..8,13,18} (7 alike) : Logic  Operator=OR  AllPortsSameDT=off  OutDataTypeStr=boolean
  AND12 : Logic  Inputs=3  AllPortsSameDT=off  OutDataTypeStr=boolean
  AND2 : Logic  Inputs=7  AllPortsSameDT=off  OutDataTypeStr=boolean
  AND3 : Logic  Inputs=7  AllPortsSameDT=off  OutDataTypeStr=boolean
  Constant : Constant  Value=SeatOccupiedSts1.SeatOccupiedSts_Empty  OutDataTypeStr=Enum:SeatOccupiedSts1
  Constant{1,3,7,17,24,27,30,33} (8 alike) : Constant  Value=IfVeSMSeStNumConfig.SeatNum7Config  OutDataTypeStr=Enum: IfVeSMSeStNumConfig
  Constant10 : Constant  Value=SeatChldLkSt.ChldLkSt_Lock  OutDataTypeStr=Enum:SeatChldLkSt
  Constant{11,19,21..23} (5 alike) : Constant  OutDataTypeStr=boolean
  Constant12 : Constant  Value=0  OutDataTypeStr=boolean
  Constant13 : Constant  Value=0  OutDataTypeStr=uint16
  Constant14 : Constant  Value=0  OutDataTypeStr=boolean
  Constant15 : Constant  Value=0  OutDataTypeStr=uint16
  Constant16 : Constant  Value=SeatChldLkSt.ChldLkSt_Lock  OutDataTypeStr=Enum:SeatChldLkSt
  Constant{2,4,8,18} (4 alike) : Constant  Value=0  OutDataTypeStr=uint8
  Constant20 : Constant  Value=SeatChldLkSt.ChldLkSt_Unlock  OutDataTypeStr=Enum:SeatChldLkSt
  Constant25 : Constant  Value=SeatOccupiedSts1.SeatOccupiedSts_Empty  OutDataTypeStr=Enum:SeatOccupiedSts1
  Constant{26,28,31,34} (4 alike) : Constant  OutDataTypeStr=uint8
  Constant29 : Constant  Value=PosRclRspStat1.PosRclRspStat_None  OutDataTypeStr=Enum:PosRclRspStat1
  Constant32 : Constant  Value=PosRclRspStat1.PosRclRspStat_None  OutDataTypeStr=Enum:PosRclRspStat1
  Constant5 : Constant  Value=IfVeSMSeStNumConfig.SeatNum7Config  OutDataTypeStr=Enum:IfVeSMSeStNumConfig
  Constant6 : Constant  Value=SeatOccupiedSts1.SeatOccupiedSts_Empty  OutDataTypeStr=Enum:SeatOccupiedSts1
  Constant9 : Constant  Value=SeatChldLkSt.ChldLkSt_Unlock  OutDataTypeStr=Enum:SeatChldLkSt
  Equal{,1..13,18..30} (27 alike) : RelationalOperator  Operator===  OutDataTypeStr=boolean  RndMeth=Simplest
  Equal14 : RelationalOperator  OutDataTypeStr=boolean  RndMeth=Simplest
  Equal15 : RelationalOperator  Operator=<  OutDataTypeStr=boolean  RndMeth=Simplest
  Equal16 : RelationalOperator  OutDataTypeStr=boolean  RndMeth=Simplest
  Equal17 : RelationalOperator  Operator=<  OutDataTypeStr=boolean  RndMeth=Simplest
  NOT{,1..3} (4 alike) : Logic  Operator=NOT  AllPortsSameDT=off  OutDataTypeStr=boolean
  Switch{,1..8} (9 alike) : Switch  Criteria=u2 > Threshold
  LugMdLtAvl : Outport
  LugMdRtAvl : Outport  Port=2
  wires:
  CommCond/1 -> AND/1
  AND/1 -> AND3/1, AND2/3
  AND2/1 -> LugMdLtAvl/1
  LugRtPosLrnd/1 -> AND3/2
  AND3/1 -> LugMdRtAvl/1
  NOT1/1 -> AND3/3
  NOT3/1 -> AND3/4
  LugMdConfig/1 -> AND/2
  ThdRwLtStOccStat/1 -> [ThdRwLtStOccStat]
  ThdRwCtStOccStat/1 -> [ThdRwCtStOccStat]
  ThdRwRtStOccStat/1 -> [ThdRwRtStOccStat]
  IfVeSMSeStNumConfig/1 -> [IfVeSMSeStNumConfig]
  Equal4/1 -> AND3/5
  Constant25/1 -> Equal4/2
  [ThdRwRtStOccStat] -> Equal4/1
  [ThdRwCtStOccStat] -> Switch/1
  Constant/1 -> Equal3/1, Equal2/2
  Equal7/1 -> Switch/2
  Equal2/1 -> AND4/1
  Equal3/1 -> AND4/2
  [ThdRwLtStOccStat] -> Equal2/1
  Constant6/1 -> Switch/3
  Constant5/1 -> Equal7/2
  Switch/1 -> Equal3/2
  [IfVeSMSeStNumConfig] -> Equal7/1
  Constant17/1 -> Equal13/2
  [IfVeSMSeStNumConfig] -> Equal13/1
  Equal13/1 -> Switch6/2
  Constant18/1 -> Switch6/3
  VeSignalLost2R_463_2L/1 -> [VeSignalLost2R_463_2L]
  AND1/1 -> NOT3/1
  Switch6/1 -> AND5/2
  AND5/1 -> NOT2/1
  [IfVeSMSeStNumConfig] -> Equal1/1
  Constant1/1 -> Equal1/2
  Equal1/1 -> Switch1/2
  Constant2/1 -> Switch1/3
  Is2LStSwAct/1 -> [Is2LStSwAct]
  Is2RStSwAct/1 -> [Is2RStSwAct]
  [Is2LStSwAct] -> AND6/1
  [Is2RStSwAct] -> AND6/2
  AND6/1 -> Switch1/1
  Switch1/1 -> AND7/2
  Is3LStSwAct/1 -> AND7/1
  AND7/1 -> NOT/1
  [VeSignalLost2R_463_2L] -> Switch6/1
  Constant4/1 -> Switch2/3
  Equal5/1 -> Switch2/2
  Constant3/1 -> Equal5/2
  [IfVeSMSeStNumConfig] -> Equal5/1
  [Is2RStSwAct] -> Switch2/1
  Switch2/1 -> AND8/2
  Is3RStSwAct/1 -> AND8/1
  AND8/1 -> NOT1/1
  [IfVeSMSeStNumConfig] -> Equal6/1
  Constant7/1 -> Equal6/2
  Equal6/1 -> Switch3/2
  Constant8/1 -> Switch3/3
  [VeSignalLost2R_463_2L] -> Switch3/1
  Switch3/1 -> AND1/2
  SecRwLtStChldLkReq/1 -> [SecRwLtStChldLkReq]
  Equal22/1 -> AND12/2
  Constant9/1 -> Equal22/1, Equal8/2
  ThdRwLtStChldLkReq/1 -> Equal22/2
  [SecRwLtStChldLkReq] -> Equal8/1
  [SecRwLtStChldLkReq] -> Equal9/1
  Constant10/1 -> Equal9/2
  SecRwLtStBkReclnUpwdDnwdPos/1 -> Equal15/1, Equal14/1
  SecRwLtStBkReclnUpwdDnwdPosV/1 -> Equal10/1
  Constant12/1 -> Equal10/2
  Constant13/1 -> Equal14/2
  AND9/1 -> AND10/1
  [KeSMSwAcsMd8SecRwLtStBkReclnUpwdDnwdPos] -> Equal15/2
  Equal10/1 -> AND10/2
  Equal15/1 -> AND9/1
  Equal14/1 -> AND9/2
  KeSMSuSecRwStBackPosDelta/1 -> [KeSMSuSecRwStBackPosDelta]
  AND10/1 -> [SecRwLtStBkReclnUpwdDnwdPosOK]
  [SecRwLtStBkReclnUpwdDnwdPosOK] -> Equal11/1
  Constant11/1 -> Equal11/2
  Equal9/1 -> AND11/1
  Equal11/1 -> AND11/2
  Equal8/1 -> AND13/2
  AND11/1 -> AND13/1
  AND13/1 -> AND12/1
  AND12/1 -> [LugLtStChldLkOK]
  AND14/1 -> [SecRwRtStBkReclnUpwdDnwdPosOK]
  Equal16/1 -> AND15/2
  Equal17/1 -> AND15/1
  Equal12/1 -> AND14/2
  [KeSMSwAcsMd9SecRwRtStBkReclnUpwdDnwdPos] -> Equal17/2
  AND15/1 -> AND14/1
  Constant15/1 -> Equal16/2
  Constant14/1 -> Equal12/2
  SecRwRtStBkReclnUpwdDnwdPosV/1 -> Equal12/1
  SecRwRtStBkReclnUpwdDnwdPos/1 -> Equal16/1, Equal17/1
  SecRwRtStChldLkReq/1 -> [SecRwRtStChldLkReq]
  AND16/1 -> AND18/1
  Equal20/1 -> AND18/2
  Equal18/1 -> AND16/2
  Equal21/1 -> AND16/1
  Constant19/1 -> Equal18/2
  Constant16/1 -> Equal21/2
  [SecRwRtStChldLkReq] -> Equal21/1
  [SecRwRtStChldLkReq] -> Equal20/1
  Constant20/1 -> Equal20/2
  [SecRwRtStBkReclnUpwdDnwdPosOK] -> Equal18/1
  AND18/1 -> [LugRtStChldLkOK], [RtStChldLkOK]
  [LugLtStChldLkOK] -> Equal/1
  Constant21/1 -> Equal/2
  Constant22/1 -> Equal19/2
  [LugRtStChldLkOK] -> Equal19/1
  [RtStChldLkOK] -> Equal24/1
  Constant23/1 -> Equal24/2
  Equal24/1 -> AND12/3
  [IfVeSMSeStNumConfig] -> Equal23/1
  Constant24/1 -> Equal23/2
  Constant26/1 -> Switch4/3
  Equal23/1 -> Switch4/2
  Equal/1 -> Switch4/1
  Constant28/1 -> Switch5/3
  Equal25/1 -> Switch5/2
  Constant27/1 -> Equal25/2
  [IfVeSMSeStNumConfig] -> Equal25/1
  Equal19/1 -> Switch5/1
  Switch5/1 -> AND3/6
  VeSignalLost3R_46C_2L/1 -> AND1/1
  VeSignalLost3L_468_2L/1 -> AND5/1
  SecRwRtStPosRclRspStat/1 -> [SecRwRtStPosRclRspStat]
  Constant29/1 -> Equal27/1, Equal26/2
  SecRwLtStPosRclRspStat/1 -> Equal26/1
  [SecRwRtStPosRclRspStat] -> Equal27/2
  Equal26/1 -> AND17/1
  Equal27/1 -> AND17/2
  Switch4/1 -> AND2/7
  NOT2/1 -> AND2/6
  NOT/1 -> AND2/5
  LugLtPosLrnd/1 -> AND2/4
  AND4/1 -> AND2/2
  Constant31/1 -> Switch7/3
  Equal28/1 -> Switch7/2
  Constant30/1 -> Equal28/2
  [IfVeSMSeStNumConfig] -> Equal28/1
  AND17/1 -> Switch7/1
  Switch7/1 -> AND2/1
  [IfVeSMSeStNumConfig] -> Equal30/1
  Equal30/1 -> Switch8/2
  Constant32/1 -> Equal29/2
  Constant33/1 -> Equal30/2
  Equal29/1 -> Switch8/1
  [SecRwRtStPosRclRspStat] -> Equal29/1
  Constant34/1 -> Switch8/3
  Switch8/1 -> AND3/7
  KeSMSwAcsMd8SecRwLtStBkReclnUpwdDnwdPos/1 -> [KeSMSwAcsMd8SecRwLtStBkReclnUpwdDnwdPos]
  KeSMSwAcsMd9SecRwRtStBkReclnUpwdDnwdPos/1 -> [KeSMSwAcsMd9SecRwRtStBkReclnUpwdDnwdPos]

== system PreCondition/PreConitionRunnable_sys/Subsystem3/LyingMd ==
  CommCond : Inport
  LyingMdConfig : Inport  Port=2
  SecRwLtStPosRclRspStat : Inport  Port=3
  SecRwRtStPosRclRspStat : Inport  Port=4
  LyingLtPosLrnd : Inport  Port=5
  LyingRtPosLrnd : Inport  Port=6
  Is2LStSwAct : Inport  Port=7
  Is2RStSwAct : Inport  Port=8
  SecRwLtStChldLkReq : Inport  Port=9
  SecRwRtStChldLkReq : Inport  Port=10
  VeSignalLost2R_463_2L : Inport  Port=11
  AND1 : Logic  Inputs=5  AllPortsSameDT=off  OutDataTypeStr=boolean
  AND2 : Logic  AllPortsSameDT=off  OutDataTypeStr=boolean
  AND3 : Logic  Inputs=6  AllPortsSameDT=off  OutDataTypeStr=boolean
  Constant1 : Constant  Value=PosRclRspStat1.PosRclRspStat_None  OutDataTypeStr=Enum:PosRclRspStat1
  Constant2 : Constant  Value=SeatChldLkSt.ChldLkSt_Unlock  OutDataTypeStr=Enum:SeatChldLkSt
  Constant3 : Constant  Value=SeatChldLkSt.ChldLkSt_Unlock  OutDataTypeStr=Enum:SeatChldLkSt
  Constant4 : Constant  Value=PosRclRspStat1.PosRclRspStat_None  OutDataTypeStr=Enum:PosRclRspStat1
  Equal{,1..2,5} (4 alike) : RelationalOperator  Operator===  OutDataTypeStr=boolean  RndMeth=Simplest
  NOT : Logic  Operator=NOT  AllPortsSameDT=off  OutDataTypeStr=boolean
  NOT1 : Logic  Operator=NOT  AllPortsSameDT=off  OutDataTypeStr=boolean
  NOT2 : Logic  Operator=NOT  AllPortsSameDT=off  OutDataTypeStr=boolean
  LyingMdLtAvl : Outport
  LyingMdRtAvl : Outport  Port=2
  wires:
  LyingMdConfig/1 -> AND2/2
  CommCond/1 -> AND2/1
  AND2/1 -> [LyingCommCond]
  SecRwLtStPosRclRspStat/1 -> Equal/1
  SecRwRtStPosRclRspStat/1 -> Equal1/2
  Constant4/1 -> Equal/2
  Constant1/1 -> Equal1/1
  Equal/1 -> AND1/2
  NOT/1 -> AND1/4
  LyingLtPosLrnd/1 -> AND1/3
  AND1/1 -> LyingMdLtAvl/1
  [LyingCommCond] -> AND1/1
  Is2LStSwAct/1 -> NOT/1
  SecRwLtStChldLkReq/1 -> Equal5/1
  Constant2/1 -> Equal5/2
  Equal5/1 -> AND1/5
  Is2RStSwAct/1 -> NOT1/1
  Equal1/1 -> AND3/2
  [LyingCommCond] -> AND3/1
  Equal2/1 -> AND3/5
  NOT1/1 -> AND3/4
  AND3/1 -> LyingMdRtAvl/1
  LyingRtPosLrnd/1 -> AND3/3
  SecRwRtStChldLkReq/1 -> Equal2/1
  Constant3/1 -> Equal2/2
  VeSignalLost2R_463_2L/1 -> NOT2/1
  NOT2/1 -> AND3/6

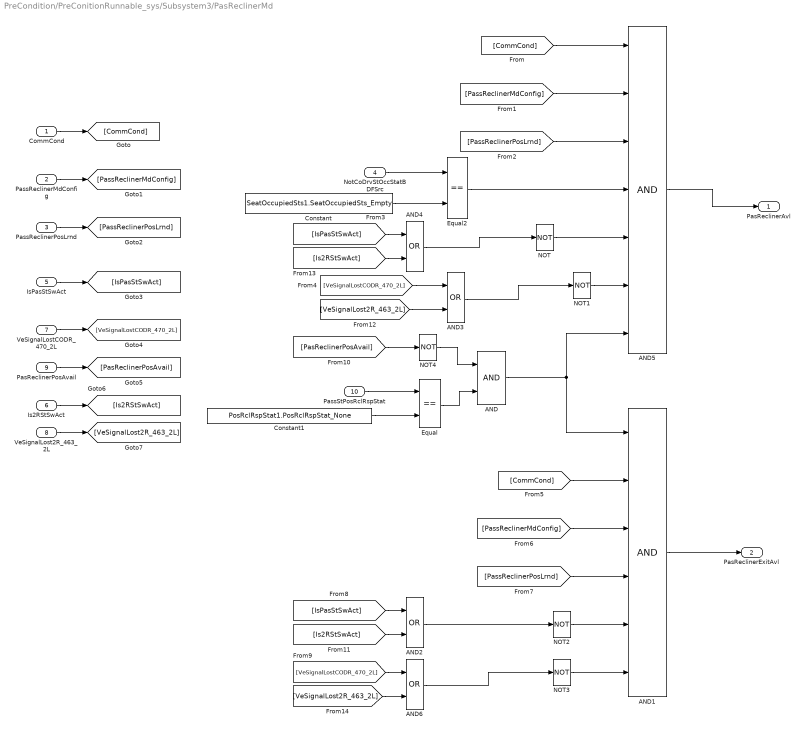
== system PreCondition/PreConitionRunnable_sys/Subsystem3/PasReclinerMd ==
  CommCond : Inport
  PassReclinerMdConfig : Inport  Port=2
  PassReclinerPosLrnd : Inport  Port=3
  NotCoDrvStOccStatBDFSrc : Inport  Port=4
  IsPasStSwAct : Inport  Port=5
  Is2RStSwAct : Inport  Port=6
  VeSignalLostCODR_470_2L : Inport  Port=7
  VeSignalLost2R_463_2L : Inport  Port=8
  PasReclinerPosAvail : Inport  Port=9
  PassStPosRclRspStat : Inport  Port=10
  AND : Logic  AllPortsSameDT=off  OutDataTypeStr=boolean
  AND1 : Logic  Inputs=6  AllPortsSameDT=off  OutDataTypeStr=boolean
  AND{2..4,6} (4 alike) : Logic  Operator=OR  AllPortsSameDT=off  OutDataTypeStr=boolean
  AND5 : Logic  Inputs=7  AllPortsSameDT=off  OutDataTypeStr=boolean
  Constant : Constant  Value=SeatOccupiedSts1.SeatOccupiedSts_Empty  OutDataTypeStr=Enum:SeatOccupiedSts1
  Constant1 : Constant  Value=PosRclRspStat1.PosRclRspStat_None  OutDataTypeStr=Enum:PosRclRspStat1
  Equal : RelationalOperator  Operator===  OutDataTypeStr=boolean  RndMeth=Simplest
  Equal2 : RelationalOperator  Operator===  OutDataTypeStr=boolean  RndMeth=Simplest
  NOT{,1..4} (5 alike) : Logic  Operator=NOT  AllPortsSameDT=off  OutDataTypeStr=boolean
  "PasReclinerAvl " : Outport
  PasReclinerExitAvl : Outport  Port=2
  wires:
  AND5/1 -> "PasReclinerAvl "/1
  NOT/1 -> AND5/5
  Constant/1 -> Equal2/2
  NotCoDrvStOccStatBDFSrc/1 -> Equal2/1
  Equal2/1 -> AND5/4
  NOT1/1 -> AND5/6
  CommCond/1 -> [CommCond]
  PassReclinerMdConfig/1 -> [PassReclinerMdConfig]
  PassReclinerPosLrnd/1 -> [PassReclinerPosLrnd]
  [CommCond] -> AND5/1
  [PassReclinerMdConfig] -> AND5/2
  [PassReclinerPosLrnd] -> AND5/3
  IsPasStSwAct/1 -> [IsPasStSwAct]
  VeSignalLostCODR_470_2L/1 -> [VeSignalLostCODR_470_2L]
  AND1/1 -> PasReclinerExitAvl/1
  PasReclinerPosAvail/1 -> [PasReclinerPosAvail]
  [PasReclinerPosAvail] -> NOT4/1
  NOT3/1 -> AND1/6
  NOT2/1 -> AND1/5
  [PassReclinerPosLrnd] -> AND1/4
  [PassReclinerMdConfig] -> AND1/3
  [CommCond] -> AND1/2
  PassStPosRclRspStat/1 -> Equal/1
  Constant1/1 -> Equal/2
  NOT4/1 -> AND/1
  Equal/1 -> AND/2
  AND/1 -> AND1/1, AND5/7
  Is2RStSwAct/1 -> [Is2RStSwAct]
  [IsPasStSwAct] -> AND4/1
  [Is2RStSwAct] -> AND2/2
  AND4/1 -> NOT/1
  VeSignalLost2R_463_2L/1 -> [VeSignalLost2R_463_2L]
  [VeSignalLostCODR_470_2L] -> AND3/1
  [VeSignalLost2R_463_2L] -> AND3/2
  AND3/1 -> NOT1/1
  [IsPasStSwAct] -> AND2/1
  [Is2RStSwAct] -> AND4/2
  [VeSignalLost2R_463_2L] -> AND6/2
  AND2/1 -> NOT2/1
  [VeSignalLostCODR_470_2L] -> AND6/1
  AND6/1 -> NOT3/1

== system PreCondition/PreConitionRunnable_sys/Subsystem3/RcvyMdAvl ==
  CommCond : Inport
  RcvyMdConfig : Inport  Port=2
  SecRwLtStPosRclRspStat : Inport  Port=3
  SecRwRtStPosRclRspStat : Inport  Port=4
  RcvyLtPosLrnd : Inport  Port=5
  RcvyRtPosLrnd : Inport  Port=6
  SecRwLtStChldLkReq : Inport  Port=7
  SecRwRtStChldLkReq : Inport  Port=8
  Is2LStSwAct : Inport  Port=9
  Is2RStSwAct : Inport  Port=10
  VeSignalLost2R_463_2L : Inport  Port=11
  AND : Logic  Inputs=5  AllPortsSameDT=off  OutDataTypeStr=boolean
  AND1 : Logic  AllPortsSameDT=off  OutDataTypeStr=boolean
  AND2 : Logic  Inputs=6  AllPortsSameDT=off  OutDataTypeStr=boolean
  Constant1 : Constant  Value=PosRclRspStat1.PosRclRspStat_None  OutDataTypeStr=Enum:PosRclRspStat1
  Constant2 : Constant  Value=SeatChldLkSt.ChldLkSt_Unlock  OutDataTypeStr=Enum:SeatChldLkSt
  Constant3 : Constant  Value=SeatChldLkSt.ChldLkSt_Unlock  OutDataTypeStr=Enum:SeatChldLkSt
  Constant4 : Constant  Value=PosRclRspStat1.PosRclRspStat_None  OutDataTypeStr=Enum:PosRclRspStat1
  Equal{,1..2,5} (4 alike) : RelationalOperator  Operator===  OutDataTypeStr=boolean  RndMeth=Simplest
  NOT : Logic  Operator=NOT  AllPortsSameDT=off  OutDataTypeStr=boolean
  NOT2 : Logic  Operator=NOT  AllPortsSameDT=off  OutDataTypeStr=boolean
  NOT4 : Logic  Operator=NOT  AllPortsSameDT=off  OutDataTypeStr=boolean
  RcvyMdLtAvl : Outport
  RcvyMdRtAvl : Outport  Port=2
  wires:
  Constant4/1 -> Equal/2
  SecRwLtStPosRclRspStat/1 -> Equal/1
  Constant2/1 -> Equal5/2
  SecRwLtStChldLkReq/1 -> Equal5/1
  RcvyLtPosLrnd/1 -> AND/2
  Equal/1 -> AND/1
  Equal5/1 -> AND/3
  CommCond/1 -> AND1/1
  RcvyMdConfig/1 -> AND1/2
  AND1/1 -> AND/4, AND2/1
  AND/1 -> RcvyMdLtAvl/1
  SecRwRtStPosRclRspStat/1 -> Equal1/1
  Constant1/1 -> Equal1/2
  Constant3/1 -> Equal2/2
  SecRwRtStChldLkReq/1 -> Equal2/1
  Equal2/1 -> AND2/4
  Equal1/1 -> AND2/2
  RcvyRtPosLrnd/1 -> AND2/3
  AND2/1 -> RcvyMdRtAvl/1
  NOT/1 -> AND/5
  NOT4/1 -> AND2/5
  NOT2/1 -> AND2/6
  VeSignalLost2R_463_2L/1 -> NOT2/1
  Is2LStSwAct/1 -> NOT/1
  Is2RStSwAct/1 -> NOT4/1
